simulink model "brakeModelTest"  (R2013b)
settings: Solver=ode45  StartTime=0.0  StopTime=100.0  MaxStep=0.01  RelTol=1e-3
InitFcn:
  | v0 = 10;
  | Rd = 0.0625;
settings Model: Creator=lasse  LastModifiedBy=lasse

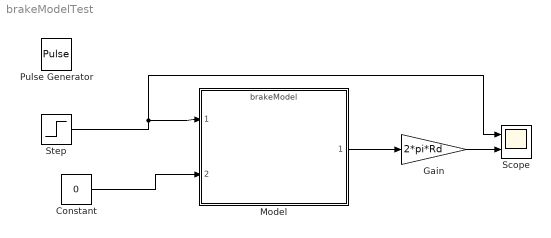
== system brakeModelTest ==
  Constant : Constant  Value=0
  Gain : Gain  Gain=2*pi*Rd
  Model : ModelReference  ModelNameDialog=brakeModel.slx  SimulationMode=Normal  ModelReferenceVersion=1.12  CopyOfModelName=brakeModel.slx  DefaultDataLogging=on
  Pulse Generator : DiscretePulseGenerator  PulseType=Time based  Period=10  PulseWidth=5
  Scope : Scope  NumInputPorts=2
      settings: TimeRange=100  YMin=0~0  YMax=100~10  MaxDataPoints=100000
  Step : Step  After=100  SampleTime=0
  wires:
  Model/1 -> Gain/1
  Gain/1 -> Scope/2
  Constant/1 -> Model/2
  Step/1 -> Scope/1, Model/1
